simulink model "Autopilot_q_full_5may_new1"  (R2020a)
settings: Solver=ode4  StartTime=0.0  StopTime=300  FixedStep=0.01  RelTol=1e-3
undefined symbols (not defined in the file or in its folder): Aero_cofficients, Atmosphere_pert, Atmospheric_model, Counter_sensor_model, Earth, error_global, flags_global, Guidance_Flags_global, INT_global, param_guidance, Payload_data, Plane_state_mode_finish_catcher_ftr_mode, Plane_state_mode_finish_catcher_fw_mode, Plane_state_mode_finish_catcher_q_mode, Plane_state_mode_finish_catcher_rtr_mode, Plane_state_store, propulsion_model, propulsion_model_int, Structural_data, Thrust_data_store, time_global, WGS84, Wind_data, Wind_model_int, Wind_pert_factor
libraries: simulink x33, aerolibactuator x15, cstblocks x3, aerolibatmos2 x2, aerolibfltsims x1, aerolibtransform2 x1, shared6dof x1
(part 4 of 10)

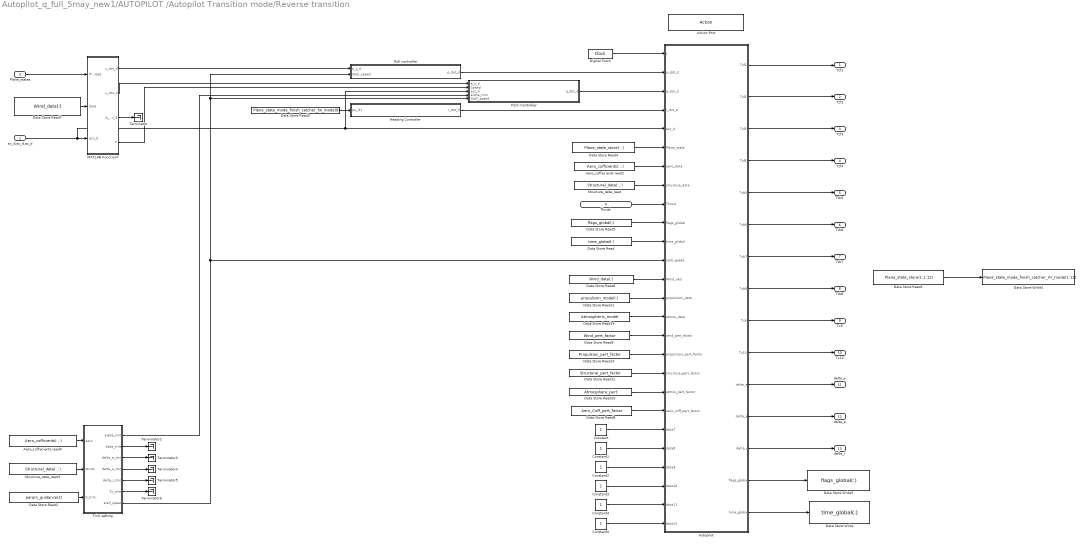
== system Autopilot_q_full_5may_new1/AUTOPILOT /Autopilot Transition mode/Reverse transition ==
  ax_d,ay_d,az_d : Inport
  Plane_states : Inport  Port=2
  Thrust : Inport  Port=3
  Action Port : ActionPort  ActionPortLabel=if { }
  Aero_coffecients read2 : DataStoreRead  Priority=1  DataStoreName=Aero_cofficients  DataStoreElements=Aero_cofficients(:,:)
  Aero_coffecients read4 : DataStoreRead  DataStoreName=Aero_cofficients  DataStoreElements=Aero_cofficients(:,:)
  Autopilot : MATLAB Function  TreatAsAtomicUnit=on
  Constant{,1..5} (6 alike) : Constant
  Data Store Read : DataStoreRead  DataStoreName=time_global  DataStoreElements=time_global(:)
  Data Store Read1 : DataStoreRead  DataStoreName=Plane_state_store  DataStoreElements=Plane_state_store(1,1:12)
  Data Store Read10 : DataStoreRead  DataStoreName=Atmosphere_pert
  Data Store Read11 : DataStoreRead  DataStoreName=propulsion_model  DataStoreElements=propulsion_model(:)
  Data Store Read12 : DataStoreRead  DataStoreName=Structural_pert_factor
  Data Store Read13 : DataStoreRead  DataStoreName=Propulsion_pert_factor
  Data Store Read14 : DataStoreRead  DataStoreName=Atmospheric_model
  Data Store Read2 : DataStoreRead  DataStoreName=param_guidance  DataStoreElements=param_guidance(2)
  Data Store Read3 : DataStoreRead  DataStoreName=Plane_state_mode_finish_catcher_fw_mode  DataStoreElements=Plane_state_mode_finish_catcher_fw_mode(9)
  Data Store Read4 : DataStoreRead  DataStoreName=Plane_state_store  DataStoreElements=Plane_state_store(:,:)
  Data Store Read5 : DataStoreRead  DataStoreName=flags_global  DataStoreElements=flags_global(:)
  Data Store Read6 : DataStoreRead  DataStoreName=Wind_data  DataStoreElements=Wind_data(:)
  Data Store Read7 : DataStoreRead  DataStoreName=Wind_data  DataStoreElements=Wind_data(:)
  Data Store Read8 : DataStoreRead  DataStoreName=Aero_Coff_pert_factor
  Data Store Read9 : DataStoreRead  DataStoreName=Wind_pert_factor
  Data Store Write : DataStoreWrite  DataStoreName=time_global  DataStoreElements=time_global(:)
  Data Store Write1 : DataStoreWrite  DataStoreName=Plane_state_mode_finish_catcher_rtr_mode  DataStoreElements=Plane_state_mode_finish_catcher_rtr_mode(1:12)
  Data Store Write5 : DataStoreWrite  DataStoreName=flags_global  DataStoreElements=flags_global(:)
  Digital Clock : DigitalClock  SampleTime=0.01
  Heading Controller : Subsystem
  MATLAB Function7 : MATLAB Function  TreatAsAtomicUnit=on
  Pitch Controller : Subsystem
  Roll controller : Subsystem
  Structure_data_read : DataStoreRead  Priority=2  DataStoreName=Structural_data  DataStoreElements=Structural_data(:,:)
  Structure_data_read3 : DataStoreRead  DataStoreName=Structural_data  DataStoreElements=Structural_data(:,:)
  Terminator{,2..6} (6 alike) : Terminator
  Trim setting : Subsystem
  Tzf1 : Outport  VectorParamsAs1DForOutWhenUnconnected=off
  Tzf2 : Outport  Port=2  VectorParamsAs1DForOutWhenUnconnected=off
  Tzf3 : Outport  Port=3  VectorParamsAs1DForOutWhenUnconnected=off
  Tzf4 : Outport  Port=4  VectorParamsAs1DForOutWhenUnconnected=off
  Tzb5 : Outport  Port=5  VectorParamsAs1DForOutWhenUnconnected=off
  Tzb6 : Outport  Port=6  VectorParamsAs1DForOutWhenUnconnected=off
  Tzb7 : Outport  Port=7  VectorParamsAs1DForOutWhenUnconnected=off
  Tzb8 : Outport  Port=8  VectorParamsAs1DForOutWhenUnconnected=off
  Tx9 : Outport  Port=9  VectorParamsAs1DForOutWhenUnconnected=off
  Tx10 : Outport  Port=10  VectorParamsAs1DForOutWhenUnconnected=off
  delta_e : Outport  Port=11  VectorParamsAs1DForOutWhenUnconnected=off
  delta_a : Outport  Port=12  VectorParamsAs1DForOutWhenUnconnected=off
  delta_r : Outport  Port=13  VectorParamsAs1DForOutWhenUnconnected=off
  wires:
  Autopilot/12(delta_a) -> delta_a/1
  MATLAB Function7/3(w_dot_d) -> Terminator/1
  Autopilot/10(Tx10) -> Tx10/1
  Roll controller/1(p_dot_d) -> Autopilot/2(p_dot_d)
  Autopilot/4(Tzf4) -> Tzf4/1
  Autopilot/1(Tzf1) -> Tzf1/1
  Autopilot/8(Tzb8) -> Tzb8/1
  Trim setting/6(Tx_trim) -> Terminator6/1
  Trim setting/2(beta_trim) -> Terminator2/1
  Heading Controller/1(r_dot_d) -> Autopilot/4(r_dot_d)
  Trim setting/3(delta_e_trim) -> Terminator3/1
  Structure_data_read3/1 -> Trim setting/2("struct ")
  Trim setting/5(delta_r_trim) -> Terminator5/1
  Autopilot/2(Tzf2) -> Tzf2/1
  Autopilot/5(Tzb5) -> Tzb5/1
  ax_d,ay_d,az_d/1 -> Pitch Controller/3(acc_d), Autopilot/5(acc_d), MATLAB Function7/3(acc_d)
  Autopilot/9(Tx9) -> Tx9/1
  Data Store Read2/1 -> Trim setting/3(V_trim)
  Autopilot/11(delta_e) -> delta_e/1
  Autopilot/6(Tzb6) -> Tzb6/1
  Autopilot/3(Tzf3) -> Tzf3/1
  Autopilot/13(delta_r) -> delta_r/1
  Aero_coffecients read4/1 -> Trim setting/1("aero ")
  Autopilot/7(Tzb7) -> Tzb7/1
  Trim setting/4(delta_a_trim) -> Terminator4/1
  Trim setting/7(stall_speed) -> Roll controller/2(Stall_speed), Pitch Controller/5(Stall_speed), Autopilot/12(stall_speed)
  Autopilot/14(flags_global) -> Data Store Write5/1
  Data Store Read5/1 -> Autopilot/10("flags_global ")
  Autopilot/15(time_global) -> Data Store Write/1
  Data Store Read/1 -> Autopilot/11("time_global ")
  Digital Clock/1 -> Autopilot/1(t)
  Data Store Read1/1 -> Data Store Write1/1
  Pitch Controller/1(q_dot_d) -> Autopilot/3(q_dot_d)
  Aero_coffecients read2/1 -> Autopilot/7(aero_data)
  Structure_data_read/1 -> Autopilot/8(structure_data)
  Thrust/1 -> Autopilot/9(Thrust)
  MATLAB Function7/1(v_dot_d) -> Roll controller/1(a_y_d)
  MATLAB Function7/2(u_dot_d) -> Pitch Controller/1(a_x_d)
  Trim setting/1(alpha_trim) -> Pitch Controller/4(alpha_trim)
  Data Store Read3/1 -> Heading Controller/1(psi_d1)
  MATLAB Function7/4(V) -> Pitch Controller/2(Speed)
  Data Store Read4/1 -> Autopilot/6(Plane_state)
  Data Store Read6/1 -> Autopilot/13(Wind_ned)
  Data Store Read7/1 -> MATLAB Function7/2(data)
  Plane_states/1 -> MATLAB Function7/1(Plane_state)
  Data Store Read11/1 -> Autopilot/14(propulsion_data)
  Data Store Read14/1 -> Autopilot/15(atmos_data)
  Data Store Read9/1 -> Autopilot/16(wind_pert_factor)
  Data Store Read13/1 -> Autopilot/17(propulsion_pert_factor)
  Data Store Read12/1 -> Autopilot/18(structure_pert_factor)
  Data Store Read10/1 -> Autopilot/19(atmos_pert_factor)
  Data Store Read8/1 -> Autopilot/20(aero_coff_pert_factor)
  Constant/1 -> Autopilot/21(data7)
  Constant1/1 -> Autopilot/22(data8)
  Constant2/1 -> Autopilot/23(data9)
  Constant3/1 -> Autopilot/24(data10)
  Constant4/1 -> Autopilot/25(data11)
  Constant5/1 -> Autopilot/26(data12)

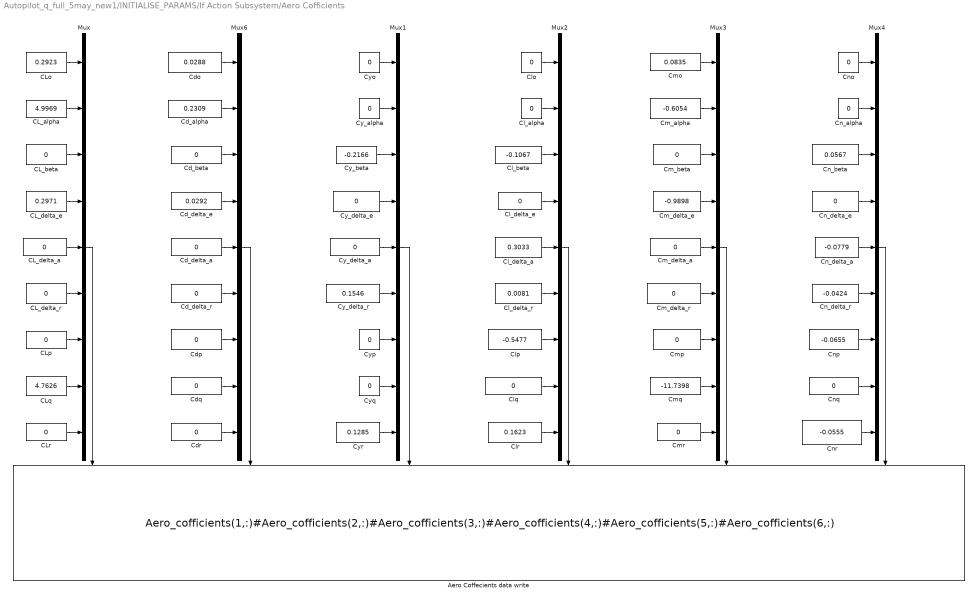
== system Autopilot_q_full_5may_new1/INITIALISE_PARAMS/If Action Subsystem/Aero Cofficients ==
  Aero Coffecients data write : DataStoreWrite  DataStoreName=Aero_cofficients  DataStoreElements=Aero_cofficients(1,:)#Aero_cofficients(2,:)#Aero_cofficients(3,:)#Aero_cofficients(4,:)#Aero_cofficients(5,:)#Aero_cofficients(6,:)
  CL_alpha : Constant  Value=4.9969
  CL_beta : Constant  Value=0
  CL_delta_a : Constant  Value=0
  CL_delta_e : Constant  Value=0.2971
  CL_delta_r : Constant  Value=0
  CLo : Constant  Value=0.2923
  CLp : Constant  Value=0
  CLq : Constant  Value=4.7626
  CLr : Constant  Value=0
  Cd_alpha : Constant  Value=0.2309
  Cd_beta : Constant  Value=0
  Cd_delta_a : Constant  Value=0
  Cd_delta_e : Constant  Value=0.0292
  Cd_delta_r : Constant  Value=0
  Cdo : Constant  Value=0.0288
  Cdp : Constant  Value=0
  Cdq : Constant  Value=0
  Cdr : Constant  Value=0
  Cl_alpha : Constant  Value=0
  Cl_beta : Constant  Value=-0.1067
  Cl_delta_a : Constant  Value=0.3033
  Cl_delta_e : Constant  Value=0
  Cl_delta_r : Constant  Value=0.0081
  Clo : Constant  Value=0
  Clp : Constant  Value=-0.5477
  Clq : Constant  Value=0
  Clr : Constant  Value=0.1623
  Cm_alpha : Constant  Value=-0.6054
  Cm_beta : Constant  Value=0
  Cm_delta_a : Constant  Value=0
  Cm_delta_e : Constant  Value=-0.9898
  Cm_delta_r : Constant  Value=0
  Cmo : Constant  Value=0.0835
  Cmp : Constant  Value=0
  Cmq : Constant  Value=-11.7398
  Cmr : Constant  Value=0
  Cn_alpha : Constant  Value=0
  Cn_beta : Constant  Value=0.0567
  Cn_delta_a : Constant  Value=-0.0779
  Cn_delta_e : Constant  Value=0
  Cn_delta_r : Constant  Value=-0.0424
  Cno : Constant  Value=0
  Cnp : Constant  Value=-0.0655
  Cnq : Constant  Value=0
  Cnr : Constant  Value=-0.0555
  Cy_alpha : Constant  Value=0
  Cy_beta : Constant  Value=-0.2166
  Cy_delta_a : Constant  Value=0
  Cy_delta_e : Constant  Value=0
  Cy_delta_r : Constant  Value=0.1546
  Cyo : Constant  Value=0
  Cyp : Constant  Value=0
  Cyq : Constant  Value=0
  Cyr : Constant  Value=0.1285
  Mux{,1..4,6} (6 alike) : Mux  Inputs=9
  wires:
  Mux/1 -> Aero Coffecients data write/1
  Cl_delta_a/1 -> Mux2/5
  Cyq/1 -> Mux1/8
  CL_beta/1 -> Mux/3
  Cdo/1 -> Mux6/1
  Cm_beta/1 -> Mux3/3
  Cy_beta/1 -> Mux1/3
  Cy_delta_e/1 -> Mux1/4
  Cm_delta_e/1 -> Mux3/4
  CLr/1 -> Mux/9
  Cnp/1 -> Mux4/7
  Cyp/1 -> Mux1/7
  CLo/1 -> Mux/1
  Cy_alpha/1 -> Mux1/2
  Cdp/1 -> Mux6/7
  CLq/1 -> Mux/8
  Cl_alpha/1 -> Mux2/2
  Cmq/1 -> Mux3/8
  Mux3/1 -> Aero Coffecients data write/5
  Cnq/1 -> Mux4/8
  Cn_delta_r/1 -> Mux4/6
  Cn_beta/1 -> Mux4/3
  Cdr/1 -> Mux6/9
  Clr/1 -> Mux2/9
  Cd_delta_a/1 -> Mux6/5
  Clq/1 -> Mux2/8
  Cn_delta_e/1 -> Mux4/4
  Clo/1 -> Mux2/1
  Cy_delta_r/1 -> Mux1/6
  Cnr/1 -> Mux4/9
  Cm_delta_r/1 -> Mux3/6
  Cyo/1 -> Mux1/1
  CL_delta_a/1 -> Mux/5
  Clp/1 -> Mux2/7
  Mux2/1 -> Aero Coffecients data write/4
  Cmp/1 -> Mux3/7
  Mux1/1 -> Aero Coffecients data write/3
  CL_delta_r/1 -> Mux/6
  Mux6/1 -> Aero Coffecients data write/2
  Cl_delta_r/1 -> Mux2/6
  Cdq/1 -> Mux6/8
  CL_delta_e/1 -> Mux/4
  Cl_beta/1 -> Mux2/3
  Cd_delta_r/1 -> Mux6/6
  Cmo/1 -> Mux3/1
  Cno/1 -> Mux4/1
  Cmr/1 -> Mux3/9
  Cyr/1 -> Mux1/9
  Cn_delta_a/1 -> Mux4/5
  Cl_delta_e/1 -> Mux2/4
  Cd_delta_e/1 -> Mux6/4
  Cd_alpha/1 -> Mux6/2
  Cm_delta_a/1 -> Mux3/5
  Cn_alpha/1 -> Mux4/2
  Cm_alpha/1 -> Mux3/2
  Cd_beta/1 -> Mux6/3
  Mux4/1 -> Aero Coffecients data write/6
  CLp/1 -> Mux/7
  CL_alpha/1 -> Mux/2
  Cy_delta_a/1 -> Mux1/5

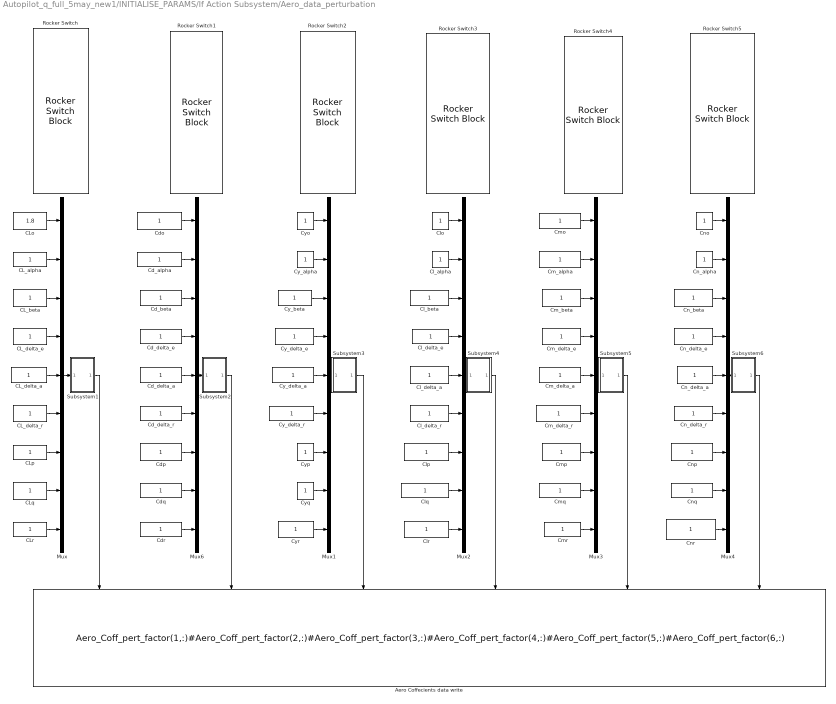
== system Autopilot_q_full_5may_new1/INITIALISE_PARAMS/If Action Subsystem/Aero_data_perturbation ==
  Aero Coffecients data write : DataStoreWrite  DataStoreName=Aero_Coff_pert_factor  DataStoreElements=Aero_Coff_pert_factor(1,:)#Aero_Coff_pert_factor(2,:)#Aero_Coff_pert_factor(3,:)#Aero_Coff_pert_factor(4,:)#Aero_Coff_pert_factor(5,:)#Aero_Coff_pert_factor(6,:)
  CL_alpha : Constant
  CL_beta : Constant
  CL_delta_a : Constant
  CL_delta_e : Constant
  CL_delta_r : Constant
  CLo : Constant  Value=1.8
  CLp : Constant
  CLq : Constant
  CLr : Constant
  Cd_alpha : Constant
  Cd_beta : Constant
  Cd_delta_a : Constant
  Cd_delta_e : Constant
  Cd_delta_r : Constant
  Cdo : Constant
  Cdp : Constant
  Cdq : Constant
  Cdr : Constant
  Cl_alpha : Constant
  Cl_beta : Constant
  Cl_delta_a : Constant
  Cl_delta_e : Constant
  Cl_delta_r : Constant
  Clo : Constant
  Clp : Constant
  Clq : Constant
  Clr : Constant
  Cm_alpha : Constant
  Cm_beta : Constant
  Cm_delta_a : Constant
  Cm_delta_e : Constant
  Cm_delta_r : Constant
  Cmo : Constant
  Cmp : Constant
  Cmq : Constant
  Cmr : Constant
  Cn_alpha : Constant
  Cn_beta : Constant
  Cn_delta_a : Constant
  Cn_delta_e : Constant
  Cn_delta_r : Constant
  Cno : Constant
  Cnp : Constant
  Cnq : Constant
  Cnr : Constant
  Cy_alpha : Constant
  Cy_beta : Constant
  Cy_delta_a : Constant
  Cy_delta_e : Constant
  Cy_delta_r : Constant
  Cyo : Constant
  Cyp : Constant
  Cyq : Constant
  Cyr : Constant
  Mux{,1..4,6} (6 alike) : Mux  Inputs=9
  Rocker Switch{,1..5} (6 alike) : RockerSwitchBlock
      settings: Values={{'Off', 'On'}, [0 1]}
  Subsystem1 : Subsystem
  Subsystem2 : Subsystem
  Subsystem3 : Subsystem
  Subsystem4 : Subsystem
  Subsystem5 : Subsystem
  Subsystem6 : Subsystem
  wires:
  CL_delta_e/1 -> Mux/4
  Cdp/1 -> Mux6/7
  Cd_alpha/1 -> Mux6/2
  Cn_delta_a/1 -> Mux4/5
  Cn_delta_e/1 -> Mux4/4
  Cmr/1 -> Mux3/9
  Cn_delta_r/1 -> Mux4/6
  Cd_delta_a/1 -> Mux6/5
  Cl_delta_e/1 -> Mux2/4
  Cd_beta/1 -> Mux6/3
  Cm_delta_a/1 -> Mux3/5
  Cd_delta_r/1 -> Mux6/6
  Cyr/1 -> Mux1/9
  Cdo/1 -> Mux6/1
  Cm_delta_e/1 -> Mux3/4
  Cyo/1 -> Mux1/1
  Cmp/1 -> Mux3/7
  Cdq/1 -> Mux6/8
  CL_delta_r/1 -> Mux/6
  Cmq/1 -> Mux3/8
  Cy_beta/1 -> Mux1/3
  Clp/1 -> Mux2/7
  CLo/1 -> Mux/1
  Cy_delta_a/1 -> Mux1/5
  CLq/1 -> Mux/8
  Cl_delta_r/1 -> Mux2/6
  CL_alpha/1 -> Mux/2
  Cnp/1 -> Mux4/7
  Cm_alpha/1 -> Mux3/2
  Cy_delta_e/1 -> Mux1/4
  Clr/1 -> Mux2/9
  Cy_alpha/1 -> Mux1/2
  Cnq/1 -> Mux4/8
  Cyp/1 -> Mux1/7
  Cnr/1 -> Mux4/9
  CLp/1 -> Mux/7
  Clq/1 -> Mux2/8
  CL_delta_a/1 -> Mux/5
  Cno/1 -> Mux4/1
  Cl_alpha/1 -> Mux2/2
  Cm_delta_r/1 -> Mux3/6
  Clo/1 -> Mux2/1
  Cdr/1 -> Mux6/9
  Cd_delta_e/1 -> Mux6/4
  Cl_delta_a/1 -> Mux2/5
  CL_beta/1 -> Mux/3
  Cmo/1 -> Mux3/1
  CLr/1 -> Mux/9
  Cyq/1 -> Mux1/8
  Cl_beta/1 -> Mux2/3
  Cy_delta_r/1 -> Mux1/6
  Cm_beta/1 -> Mux3/3
  Cn_beta/1 -> Mux4/3
  Cn_alpha/1 -> Mux4/2
  Mux/1 -> Subsystem1/1(In1)
  Subsystem1/1(Out1) -> Aero Coffecients data write/1
  Mux6/1 -> Subsystem2/1(In1)
  Subsystem2/1(Out1) -> Aero Coffecients data write/2
  Mux1/1 -> Subsystem3/1(In1)
  Mux2/1 -> Subsystem4/1(In1)
  Mux3/1 -> Subsystem5/1(In1)
  Mux4/1 -> Subsystem6/1(In1)
  Subsystem3/1(Out1) -> Aero Coffecients data write/3
  Subsystem4/1(Out1) -> Aero Coffecients data write/4
  Subsystem5/1(Out1) -> Aero Coffecients data write/5
  Subsystem6/1(Out1) -> Aero Coffecients data write/6

== system Autopilot_q_full_5may_new1/INITIALISE_PARAMS/If Action Subsystem/Atmosphere_pert ==
  note: Temp
  note: density
  note: a
  note: p
  Constant{,1..3} (4 alike) : Constant
  Data Store Write : DataStoreWrite  DataStoreName=Atmosphere_pert  DataStoreElements=Atmosphere_pert(:)
  Mux : Mux
  Rocker Switch : RockerSwitchBlock
      settings: Values={{'Off', 'On'}, [0 1]}
  Subsystem1 : Subsystem
  wires:
  Subsystem1/1(Out1) -> Data Store Write/1
  Constant/1 -> Mux/1
  Mux/1 -> Subsystem1/1(In1)
  Constant1/1 -> Mux/2
  Constant2/1 -> Mux/3
  Constant3/1 -> Mux/4

== system Autopilot_q_full_5may_new1/INITIALISE_PARAMS/If Action Subsystem/Atmospheric model ==
  Abs : Abs
  Constant : Constant  Value=0.1
  Data Store Write : DataStoreWrite  DataStoreName=Atmospheric_model  DataStoreElements=Atmospheric_model(:)
  ISA Atmosphere Model : aerolibatmos2/ISA Atmosphere Model  custom=off  g=9.80665  gamma=1.4  R=287.0531  L=0.0065  h_trop=11000  h_strat=20000  rho0=1.225  P0=101325  T0=288.15  h0=0
  Mux : Mux
  Scope{1..2,4..5} (4 alike) : Scope
  wires:
  ISA Atmosphere Model/4 -> Scope2/1, Mux/4
  ISA Atmosphere Model/1 -> Scope1/1, Mux/1
  ISA Atmosphere Model/2 -> Mux/2, Scope4/1
  ISA Atmosphere Model/3 -> Mux/3, Scope5/1
  Abs/1 -> ISA Atmosphere Model/1
  Mux/1 -> Data Store Write/1
  Constant/1 -> Abs/1

== system Autopilot_q_full_5may_new1/INITIALISE_PARAMS/If Action Subsystem/INT_global ==
  INT_GLOBAL : DataStoreWrite  DataStoreName=INT_global  DataStoreElements=INT_global(1)#INT_global(2)#INT_global(3)#INT_global(4)#INT_global(5)#INT_global(6)#INT_global(7)#INT_global(8)#INT_global(9)#INT_global(10)#INT_global(11)#INT_global(12)#INT_global(13)#INT_global(14)
  INT_VX : Constant  Value=0
  INT_VY : Constant  Value=0
  INT_VZ : Constant  Value=0
  INT_X : Constant  Value=0
  INT_Y : Constant  Value=0
  INT_Z : Constant  Value=0
  INT_alpha : Constant  Value=0
  INT_beta : Constant  Value=0
  INT_p : Constant  Value=0
  INT_phi : Constant  Value=0
  INT_psi : Constant  Value=0
  INT_q : Constant  Value=0
  INT_r : Constant  Value=0
  INT_theta : Constant  Value=0
  wires:
  INT_VX/1 -> INT_GLOBAL/4
  INT_r/1 -> INT_GLOBAL/12
  INT_Y/1 -> INT_GLOBAL/2
  INT_q/1 -> INT_GLOBAL/11
  INT_beta/1 -> INT_GLOBAL/14
  INT_Z/1 -> INT_GLOBAL/3
  INT_VZ/1 -> INT_GLOBAL/6
  INT_phi/1 -> INT_GLOBAL/7
  INT_X/1 -> INT_GLOBAL/1
  INT_p/1 -> INT_GLOBAL/10
  INT_VY/1 -> INT_GLOBAL/5
  INT_theta/1 -> INT_GLOBAL/8
  INT_alpha/1 -> INT_GLOBAL/13
  INT_psi/1 -> INT_GLOBAL/9

== system Autopilot_q_full_5may_new1/INITIALISE_PARAMS/If Action Subsystem/Params ==
  Cruise_speed : Constant  Value=25
  lim_pos : Constant  Value=0.001
  lim_vel : Constant  Value=0.001
  loiter radius : Constant  Value=60
  time store write 1 : DataStoreWrite  DataStoreName=param_guidance  DataStoreElements=param_guidance(1)#param_guidance(2)#param_guidance(3)#param_guidance(4)
  wires:
  Cruise_speed/1 -> time store write 1/2
  loiter radius/1 -> time store write 1/1
  lim_vel/1 -> time store write 1/4
  lim_pos/1 -> time store write 1/3

== system Autopilot_q_full_5may_new1/INITIALISE_PARAMS/If Action Subsystem/Payload_data ==
  note: Payload Model on off
  Constant : Constant  Value=0
  Data Store Write : DataStoreWrite  DataStoreName=Payload_data  DataStoreElements=Payload_data(1)
  Rocker Switch : RockerSwitchBlock
      settings: Values={{'Off', 'On'}, [0 1]}
  wires:
  Constant/1 -> Data Store Write/1

== system Autopilot_q_full_5may_new1/INITIALISE_PARAMS/If Action Subsystem/Propulsion_Model ==
  Data Store Write : DataStoreWrite  DataStoreName=propulsion_model_int  DataStoreElements=propulsion_model_int(:)
  Data Store Write1 : DataStoreWrite  DataStoreName=propulsion_model  DataStoreElements=propulsion_model(:)
  Mux : Mux
  PUSHER Propeller drag factor : Constant  Value=1.9899*10^-8
  PUSHER Propeller thrust factor : Constant  Value=6.679*10^-7
  VTOL Propeller drag factor : Constant  Value=1.8928*10^-8
  VTOL Propeller thrust factor : Constant  Value=5.6143*10^-7
  wires:
  VTOL Propeller thrust factor/1 -> Mux/1
  VTOL Propeller drag factor/1 -> Mux/2
  Mux/1 -> Data Store Write1/1, Data Store Write/1
  PUSHER Propeller thrust factor/1 -> Mux/3
  PUSHER Propeller drag factor/1 -> Mux/4

== system Autopilot_q_full_5may_new1/INITIALISE_PARAMS/If Action Subsystem/Propulsion_data_pert ==
  note: b_vtol
  note: d_vtol
  note: d_pusher
  note: b_pusher
  Constant{,1..3} (4 alike) : Constant
  Data Store Write : DataStoreWrite  DataStoreName=Propulsion_pert_factor  DataStoreElements=Propulsion_pert_factor(1:2)#Propulsion_pert_factor(3:4)
  Mux : Mux  Inputs=2
  Mux1 : Mux  Inputs=2
  Rocker Switch : RockerSwitchBlock
      settings: Values={{'Off', 'On'}, [0 1]}
  Rocker Switch1 : RockerSwitchBlock
      settings: Values={{'Off', 'On'}, [0 1]}
  Subsystem1 : Subsystem
  Subsystem2 : Subsystem
  wires:
  Constant/1 -> Mux/1
  Mux/1 -> Subsystem1/1(In1)
  Constant1/1 -> Mux/2
  Subsystem1/1(Out1) -> Data Store Write/1
  Constant3/1 -> Mux1/2
  Mux1/1 -> Subsystem2/1(In1)
  Constant2/1 -> Mux1/1
  Subsystem2/1(Out1) -> Data Store Write/2

== system Autopilot_q_full_5may_new1/INITIALISE_PARAMS/If Action Subsystem/Structure_data ==
  Ixx : Constant  Value=0.6275
  Ixy : Constant  Value=0
  Ixz : Constant  Value=0
  Iyy : Constant  Value=0.564
  Iyz : Constant  Value=0
  Izz : Constant  Value=1.176
  Mass : Constant  Value=5
  Structure data write1 : DataStoreWrite  DataStoreName=Structural_data  DataStoreElements=Structural_data(1,1)#Structural_data(1,2)#Structural_data(1,3)#Structural_data(1,4)#Structural_data(1,5)#Structural_data(1,6)#Structural_data(1,7)#Structural_data(1,8)#Structural_data(1,9)#Structural_data(1,10)#Structural_data(1,11)#Structural_data(1,12)#Structural_data(1,13)#Structural_data(1,14)#Structural_data(1,15)#Structural_data(1,16)#Structural_data(1,17)#Structural_data(1,18)#Structural_data(1,19)#Structural_data(1,20)#Structural_data(1,21)#Structural_data(1,22)#Structural_data(1,23)#Structural_data(1,24)
  b : Constant  Value=2.2
  c : Constant  Value=0.2104
  mb : Constant  Value=0
  s : Constant  Value=0.4626
  x1 : Constant  Value=743/2000
  x2 : Constant  Value=-743/2000
  y1 : Constant  Value=-838/1000
  y10 : Constant  Value=0
  y2 : Constant  Value=-838/2000
  y3 : Constant  Value=838/2000
  y4 : Constant  Value=838/1000
  y5 : Constant  Value=-838/1000
  y6 : Constant  Value=-838/2000
  y7 : Constant  Value=838/2000
  y8 : Constant  Value=838/1000
  y9 : Constant  Value=0.0
  z1 : Constant  Value=0
  wires:
  y5/1 -> Structure data write1/17
  Ixz/1 -> Structure data write1/9
  y6/1 -> Structure data write1/18
  y3/1 -> Structure data write1/15
  s/1 -> Structure data write1/4
  b/1 -> Structure data write1/3
  z1/1 -> Structure data write1/23
  y8/1 -> Structure data write1/20
  Mass/1 -> Structure data write1/1
  x2/1 -> Structure data write1/12
  y2/1 -> Structure data write1/14
  y10/1 -> Structure data write1/22
  y9/1 -> Structure data write1/21
  Iyy/1 -> Structure data write1/6
  c/1 -> Structure data write1/2
  mb/1 -> Structure data write1/24
  Ixx/1 -> Structure data write1/5
  x1/1 -> Structure data write1/11
  y4/1 -> Structure data write1/16
  Iyz/1 -> Structure data write1/10
  Izz/1 -> Structure data write1/7
  y7/1 -> Structure data write1/19
  Ixy/1 -> Structure data write1/8
  y1/1 -> Structure data write1/13

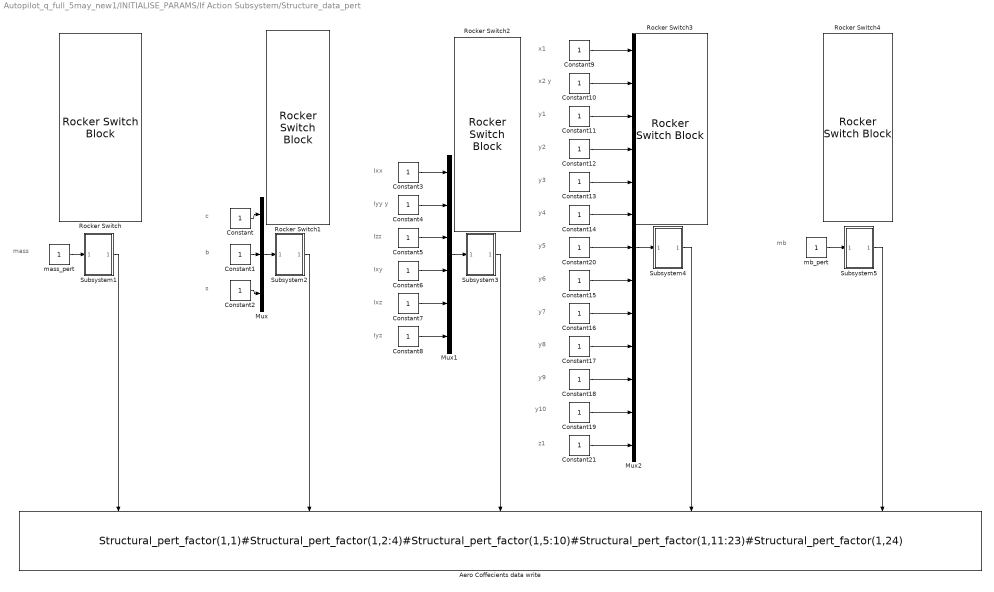
== system Autopilot_q_full_5may_new1/INITIALISE_PARAMS/If Action Subsystem/Structure_data_pert ==
  note: c
  note: b
  note: s
  note: Ixx
  note: Iyy y
  note: Izz
  note: Ixy
  note: Ixz
  note: Iyz
  note: mass
  note: y4
  note: y2
  note: y3
  note: x2 y
  note: x1
  note: y1
  note: y6
  note: y7
  note: y8
  note: y5
  note: z1
  note: y10
  note: y9
  note: mb
  Aero Coffecients data write : DataStoreWrite  DataStoreName=Structural_pert_factor  DataStoreElements=Structural_pert_factor(1,1)#Structural_pert_factor(1,2:4)#Structural_pert_factor(1,5:10)#Structural_pert_factor(1,11:23)#Structural_pert_factor(1,24)
  Constant{,1..21} (22 alike) : Constant
  Mux : Mux  Inputs=3
  Mux1 : Mux  Inputs=6
  Mux2 : Mux  Inputs=13
  Rocker Switch{,1..4} (5 alike) : RockerSwitchBlock
      settings: Values={{'Off', 'On'}, [0 1]}
  Subsystem1 : Subsystem
  Subsystem2 : Subsystem
  Subsystem3 : Subsystem
  Subsystem4 : Subsystem
  Subsystem5 : Subsystem
  mass_pert : Constant
  mb_pert : Constant
  wires:
  Mux1/1 -> Subsystem3/1(In1)
  Subsystem1/1(Out1) -> Aero Coffecients data write/1
  Subsystem5/1(Out1) -> Aero Coffecients data write/5
  Subsystem4/1(Out1) -> Aero Coffecients data write/4
  Subsystem3/1(Out1) -> Aero Coffecients data write/3
  Subsystem2/1(Out1) -> Aero Coffecients data write/2
  mass_pert/1 -> Subsystem1/1(In1)
  Mux/1 -> Subsystem2/1(In1)
  Constant/1 -> Mux/1
  Constant1/1 -> Mux/2
  Constant2/1 -> Mux/3
  Constant3/1 -> Mux1/1
  Constant4/1 -> Mux1/2
  Constant5/1 -> Mux1/3
  Constant6/1 -> Mux1/4
  Constant7/1 -> Mux1/5
  Constant8/1 -> Mux1/6
  Constant14/1 -> Mux2/6
  Constant9/1 -> Mux2/1
  Constant13/1 -> Mux2/5
  Constant11/1 -> Mux2/3
  Constant10/1 -> Mux2/2
  Constant12/1 -> Mux2/4
  Mux2/1 -> Subsystem4/1(In1)
  Constant20/1 -> Mux2/7
  Constant17/1 -> Mux2/10
  Constant15/1 -> Mux2/8
  Constant16/1 -> Mux2/9
  Constant19/1 -> Mux2/12
  Constant18/1 -> Mux2/11
  mb_pert/1 -> Subsystem5/1(In1)
  Constant21/1 -> Mux2/13

== system Autopilot_q_full_5may_new1/INITIALISE_PARAMS/If Action Subsystem/Time_global ==
  note: Initial lift off hover
  note: Vertical lift off
  note: Hover
  note: Cruise/Loiter , All fixed wing here
  note: Reverse Transition
  note: Hover
  note: Vertical Landing
  note: Forward Transition
  tf0 : Constant  Value=0
  tf1 : Constant  Value=0
  tf2 : Constant  Value=20
  tf3 : Constant  Value=22
  tf4 : Constant  Value=30
  tf5 : Constant  Value=50
  tf6 : Constant  Value=70
  tf7 : Constant  Value=72
  tf8 : Constant  Value=92
  "time store write " : DataStoreWrite  DataStoreName=time_global  DataStoreElements=time_global(1)#time_global(2)#time_global(3)#time_global(4)#time_global(5)#time_global(6)#time_global(7)#time_global(8)#time_global(9)
  wires:
  tf4/1 -> "time store write "/5
  tf8/1 -> "time store write "/9
  tf1/1 -> "time store write "/2
  tf6/1 -> "time store write "/7
  tf2/1 -> "time store write "/3
  tf5/1 -> "time store write "/6
  tf0/1 -> "time store write "/1
  tf7/1 -> "time store write "/8
  tf3/1 -> "time store write "/4

== system Autopilot_q_full_5may_new1/INITIALISE_PARAMS/If Action Subsystem/Wind_Model ==
  note: turb_on_off<50 m
  note: VN
  note: VE
  note: VD
  note: turb_on_off- 50-600 m
  note: turb_on_off>600 m
  note: turb_on_off<50 m
  note: turb_on_off- 50-600 m
  note: turb_on_off>600 m
  Constant4 : Constant  Value=0
  Constant5 : Constant  Value=0
  Constant6 : Constant  Value=0
  Data Store Write : DataStoreWrite  DataStoreName=Wind_model_int  DataStoreElements=Wind_model_int(1:3)
  Data Store Write1 : DataStoreWrite  DataStoreName=Wind_model_int  DataStoreElements=Wind_model_int(4:10)
  Moderate_turbulence_50 : RockerSwitchBlock
      settings: Values={{'Off', 'On'}, [0 1]}
  Mux : Mux  Inputs=3
  Mux1 : Mux  Inputs=7
  Rocker Switch : RockerSwitchBlock
      settings: Values={{'Off', 'On'}, [0 1]}
  Rocker Switch1 : RockerSwitchBlock
      settings: Values={{'Off', 'On'}, [0 1]}
  Rocker Switch2 : RockerSwitchBlock
      settings: Values={{'Off', 'On'}, [0 1]}
  light_turb_2 : Constant  Value=0
  light_turb_50 : Constant
  light_turb_600 : Constant
  light_turbulence_50 : RockerSwitchBlock
      settings: Values={{'Off', 'On'}, [0 1]}
  light_turbulence_600 : RockerSwitchBlock
      settings: Values={{'Off', 'On'}, [0 1]}
  mod_turb_50 : Constant  Value=0
  mod_turb_600 : Constant  Value=0
  moderate_turbulence_600 : RockerSwitchBlock
      settings: Values={{'Off', 'On'}, [0 1]}
  turb_50 : Constant  Value=0
  turb_50_600 : Constant  Value=0
  wires:
  Constant4/1 -> Mux/1
  Constant5/1 -> Mux/2
  Constant6/1 -> Mux/3
  Mux/1 -> Data Store Write/1
  light_turb_600/1 -> Mux1/3
  light_turb_50/1 -> Mux1/1
  mod_turb_50/1 -> Mux1/2
  mod_turb_600/1 -> Mux1/4
  Mux1/1 -> Data Store Write1/1
  turb_50_600/1 -> Mux1/6
  light_turb_2/1 -> Mux1/7
  turb_50/1 -> Mux1/5

== system Autopilot_q_full_5may_new1/INITIALISE_PARAMS/If Action Subsystem/Wind_data_pert ==
  note: V_N
  note: V_E
  note: V_D
  Constant : Constant
  Constant1 : Constant
  Constant2 : Constant
  Data Store Write : DataStoreWrite  DataStoreName=Wind_pert_factor  DataStoreElements=Wind_pert_factor(:)
  Mux : Mux  Inputs=3
  Rocker Switch : RockerSwitchBlock
      settings: Values={{'Off', 'On'}, [0 1]}
  Subsystem1 : Subsystem
  wires:
  Subsystem1/1(Out1) -> Data Store Write/1
  Mux/1 -> Subsystem1/1(In1)
  Constant/1 -> Mux/1
  Constant1/1 -> Mux/2
  Constant2/1 -> Mux/3

== system Autopilot_q_full_5may_new1/INITIALISE_PARAMS/If Action Subsystem/error_global ==
  ERROR_GLOBAL : DataStoreWrite  DataStoreName=error_global  DataStoreElements=error_global(1)#error_global(2)#error_global(3)#error_global(4)#error_global(5)#error_global(6)
  error_VX : Constant  Value=0
  error_VY : Constant  Value=0
  error_VZ : Constant  Value=0
  error_X : Constant  Value=0
  error_Y : Constant  Value=0
  error_Z : Constant  Value=0
  wires:
  error_Y/1 -> ERROR_GLOBAL/2
  error_VY/1 -> ERROR_GLOBAL/5
  error_X/1 -> ERROR_GLOBAL/1
  error_VZ/1 -> ERROR_GLOBAL/6
  error_Z/1 -> ERROR_GLOBAL/3
  error_VX/1 -> ERROR_GLOBAL/4

== system Autopilot_q_full_5may_new1/INITIALISE_PARAMS/If Action Subsystem/flags_global ==
  Fixed_wing_mode : Constant  Value=0
  Transition_mode : Constant  Value=0
  all_initial_check_ok : Constant
  brake_mode : Constant  Value=0
  default_mode : Constant
  fail_cruise_mode : Constant  Value=0
  fail_hover_mode : Constant  Value=0
  fail_safe_mode : Constant  Value=0
  fail_safe_mode_2 : Constant  Value=0
  fail_safe_mode_hover : Constant  Value=0
  fail_safe_mode_land : Constant  Value=0
  "flag store write " : DataStoreWrite  DataStoreName=flags_global  DataStoreElements=flags_global(1)#flags_global(2)#flags_global(3)#flags_global(4)#flags_global(5)#flags_global(6)#flags_global(7)#flags_global(8)#flags_global(9)#flags_global(10)#flags_global(11)#flags_global(12)#flags_global(13)#flags_global(14)#flags_global(15)#flags_global(16)#flags_global(17)#flags_global(18)#flags_global(19)#flags_global(20)#flags_global(21)#flags_global(22)#flags_global(23)#flags_global(24)#flags_global(25)#flags_global(26)
  flag_Forward_transition : Constant  Value=0
  flag_circle_mode : Constant  Value=0
  flag_initial_lift_off_hover : Constant
  flag_reverse_transition : Constant  Value=0
  flag_vertical_landing : Constant  Value=0
  flag_vertical_takeoff : Constant  Value=0
  one_time_initial_circle_mode : Constant
  one_time_initial_cruise_mode : Constant
  one_time_initial_forward_transition : Constant
  one_time_initial_hover_mode : Constant
  one_time_initial_lift_off_hover : Constant
  one_time_initial_reverse_transition : Constant
  one_time_initial_vertical_landing : Constant
  one_time_initial_vertical_takeoff : Constant
  quad_mode : Constant
  wires:
  one_time_initial_hover_mode/1 -> "flag store write "/18
  one_time_initial_vertical_landing/1 -> "flag store write "/21
  one_time_initial_reverse_transition/1 -> "flag store write "/26
  flag_reverse_transition/1 -> "flag store write "/24
  one_time_initial_forward_transition/1 -> "flag store write "/25
  one_time_initial_circle_mode/1 -> "flag store write "/20
  all_initial_check_ok/1 -> "flag store write "/1
  fail_hover_mode/1 -> "flag store write "/12
  Transition_mode/1 -> "flag store write "/4
  one_time_initial_lift_off_hover/1 -> "flag store write "/16
  fail_safe_mode_hover/1 -> "flag store write "/7
  brake_mode/1 -> "flag store write "/22
  one_time_initial_vertical_takeoff/1 -> "flag store write "/17
  flag_circle_mode/1 -> "flag store write "/13
  flag_initial_lift_off_hover/1 -> "flag store write "/10
  quad_mode/1 -> "flag store write "/3
  one_time_initial_cruise_mode/1 -> "flag store write "/19
  fail_safe_mode_2/1 -> "flag store write "/9
  flag_vertical_takeoff/1 -> "flag store write "/11
  fail_safe_mode/1 -> "flag store write "/6
  fail_cruise_mode/1 -> "flag store write "/14
  flag_Forward_transition/1 -> "flag store write "/23
  Fixed_wing_mode/1 -> "flag store write "/5
  default_mode/1 -> "flag store write "/2
  flag_vertical_landing/1 -> "flag store write "/15
  fail_safe_mode_land/1 -> "flag store write "/8

== system Autopilot_q_full_5may_new1/Wind_Model/System3/Subsystem1 ==
  i : Inport
  num : Inport  Port=2
  den : Inport  Port=3
  Derivative : Derivative
  Integrator : Integrator
  Integrator1 : Integrator
  MATLAB Function : MATLAB Function  TreatAsAtomicUnit=on
  Scope : Scope
  Scope1 : Scope
  Scope2 : Scope
  v_pert : Outport  VectorParamsAs1DForOutWhenUnconnected=off
  wires:
  Derivative/1 -> MATLAB Function/2(ii), Scope/1
  Integrator1/1 -> Scope2/1, v_pert/1, MATLAB Function/5(y)
  MATLAB Function/1(yyy) -> Integrator/1
  Integrator/1 -> Integrator1/1, MATLAB Function/6(yy)
  i/1 -> MATLAB Function/1(i), Derivative/1, Scope1/1
  num/1 -> MATLAB Function/3(num)
  den/1 -> MATLAB Function/4(den)

== system Autopilot_q_full_5may_new1/Wind_Model/System3/Subsystem4 ==
  i : Inport
  num : Inport  Port=2
  den : Inport  Port=3
  Integrator : Integrator
  MATLAB Function : MATLAB Function  TreatAsAtomicUnit=on
  Scope2 : Scope
  u_pert : Outport  VectorParamsAs1DForOutWhenUnconnected=off
  wires:
  den/1 -> MATLAB Function/3(den)
  num/1 -> MATLAB Function/2(num)
  i/1 -> MATLAB Function/1(i)
  Integrator/1 -> Scope2/1, u_pert/1, MATLAB Function/4(y)
  MATLAB Function/1(yy) -> Integrator/1

== system Autopilot_q_full_5may_new1/Wind_Model/System3/Subsystem5 ==
  i : Inport
  num : Inport  Port=2
  den : Inport  Port=3
  Band-Limited White Noise : simulink/Sources/Band-Limited White Noise  Cov=[0.001]  Ts=0.01  seed=[23341]
  Gain : Gain  Gain=0.01
  Integrator : Integrator
  Integrator1 : Integrator
  MATLAB Function : MATLAB Function  TreatAsAtomicUnit=on
  Scope2 : Scope
  Subtract : Sum  Inputs=+-
  w_pert : Outport  VectorParamsAs1DForOutWhenUnconnected=off
  wires:
  MATLAB Function/1(yyy) -> Integrator/1
  i/1 -> MATLAB Function/1(i), Subtract/1
  Integrator1/1 -> Scope2/1, w_pert/1, MATLAB Function/5(y)
  Integrator/1 -> Integrator1/1, MATLAB Function/6(yy)
  den/1 -> MATLAB Function/4(den)
  num/1 -> MATLAB Function/3(num)
  Subtract/1 -> Gain/1
  Gain/1 -> MATLAB Function/2(ii)
  Band-Limited White Noise/1 -> Subtract/2

== system Autopilot_q_full_5may_new1/AUTOPILOT /Autopilot Transition mode/Forward transition/Heading Controller ==
  "time " : Inport
  psi_d1 : Inport  Port=2
  Demux1 : Demux  Outputs=2
  Gain{,1..3} (4 alike) : Gain  Gain=57.3
  MATLAB Function : MATLAB Function  TreatAsAtomicUnit=on
  MATLAB Function5 : MATLAB Function  TreatAsAtomicUnit=on
  MATLAB Function6 : MATLAB Function  TreatAsAtomicUnit=on
  PID Controller : simulink/Continuous/PID Controller  Controller=PID  TimeDomain=Discrete-time  SampleTime=0.01  IntegratorMethod=Forward Euler  FilterMethod=Forward Euler  Form=Parallel  UseFilter=on  ControllerParametersSource=internal  P=0.33  I=0  D=0  N=100  InitialConditionSource=internal  InitialConditionForIntegrator=0  InitialConditionForFilter=0  ExternalReset=none  LimitOutput=off  UpperSaturationLimit=inf  LowerSaturationLimit=-inf  LinearizeAsGain=on  AntiWindupMode=none  Kb=1  TrackingMode=off  Kt=1  PParamMin=[]  PParamMax=[]  IParamMin=[]  IParamMax=[]  DParamMin=[]  DParamMax=[]  NParamMin=[]  NParamMax=[]  KbParamMin=[]  KbParamMax=[]  KtParamMin=[]  KtParamMax=[]  POutMin=[]  POutMax=[]  IOutMin=[]  IOutMax=[]  DOutMin=[]  DOutMax=[]  NOutMin=[]  NOutMax=[]  KbOutMin=[]  KbOutMax=[]  KtOutMin=[]  KtOutMax=[]  IntegratorOutMin=[]  IntegratorOutMax=[]  FilterOutMin=[]  FilterOutMax=[]  SumOutMin=[]  SumOutMax=[]  SumI1OutMin=[]  SumI1OutMax=[]  SumI2OutMin=[]  SumI2OutMax=[]  SumI3OutMin=[]  SumI3OutMax=[]  SumDOutMin=[]  SumDOutMax=[]  SaturationOutMin=[]  SaturationOutMax=[]  IntegratorContinuousStateAttributes=''  IntegratorStateMustResolveToSignalObject=off  IntegratorRTWStateStorageClass=Auto  FilterContinuousStateAttributes=''  FilterStateMustResolveToSignalObject=off  FilterRTWStateStorageClass=Auto  DifferentiatorICPrevScaledInput=0  DifferentiatorOutMin=[]  DifferentiatorOutMax=[]  FilterDiffOutCoefMin=[]  FilterDiffOutCoefMax=[]  SumDenOutMin=[]  SumDenOutMax=[]  SumNumOutMin=[]  SumNumOutMax=[]  ReciprocalOutMin=[]  ReciprocalOutMax=[]  DivideOutMin=[]  DivideOutMax=[]  TunerSelectOption=Transfer Function Based (PID Tuner App)
  PID Controller (2DOF)5 : simulink/Continuous/PID Controller (2DOF)  Controller=PID  TimeDomain=Discrete-time  SampleTime=0.01  IntegratorMethod=Forward Euler  FilterMethod=Forward Euler  Form=Parallel  UseFilter=on  ControllerParametersSource=internal  P=1.0  I=0.5  D=0  N=100  b=1  c=1  InitialConditionSource=internal  InitialConditionForIntegrator=0  InitialConditionForFilter=0  ExternalReset=none  LimitOutput=off  UpperSaturationLimit=inf  LowerSaturationLimit=-inf  LinearizeAsGain=on  AntiWindupMode=none  Kb=1  TrackingMode=off  Kt=1  PParamMin=[]  PParamMax=[]  IParamMin=[]  IParamMax=[]  DParamMin=[]  DParamMax=[]  NParamMin=[]  NParamMax=[]  bParamMin=[]  bParamMax=[]  cParamMin=[]  cParamMax=[]  KbParamMin=[]  KbParamMax=[]  KtParamMin=[]  KtParamMax=[]  POutMin=[]  POutMax=[]  IOutMin=[]  IOutMax=[]  DOutMin=[]  DOutMax=[]  NOutMin=[]  NOutMax=[]  bOutMin=[]  bOutMax=[]  cOutMin=[]  cOutMax=[]  KbOutMin=[]  KbOutMax=[]  KtOutMin=[]  KtOutMax=[]  IntegratorOutMin=[]  IntegratorOutMax=[]  FilterOutMin=[]  FilterOutMax=[]  SumOutMin=[]  SumOutMax=[]  Sum1OutMin=[]  Sum1OutMax=[]  Sum2OutMin=[]  Sum2OutMax=[]  Sum3OutMin=[]  Sum3OutMax=[]  SumI1OutMin=[]  SumI1OutMax=[]  SumI2OutMin=[]  SumI2OutMax=[]  SumI3OutMin=[]  SumI3OutMax=[]  SumDOutMin=[]  SumDOutMax=[]  SaturationOutMin=[]  SaturationOutMax=[]  IntegratorContinuousStateAttributes=''  IntegratorStateMustResolveToSignalObject=off  IntegratorRTWStateStorageClass=Auto  FilterContinuousStateAttributes=''  FilterStateMustResolveToSignalObject=off  FilterRTWStateStorageClass=Auto  DifferentiatorICPrevScaledInput=0  DifferentiatorOutMin=[]  DifferentiatorOutMax=[]  FilterDiffOutCoefMin=[]  FilterDiffOutCoefMax=[]  SumDenOutMin=[]  SumDenOutMax=[]  SumNumOutMin=[]  SumNumOutMax=[]  ReciprocalOutMin=[]  ReciprocalOutMax=[]  DivideOutMin=[]  DivideOutMax=[]  TunerSelectOption=Transfer Function Based (PID Tuner App)
  Scope : Scope  NumInputPorts=2
  Scope1 : Scope  NumInputPorts=2
  p,q,r,phi,theta,psi : DataStoreRead  DataStoreName=Plane_state_store  DataStoreElements=Plane_state_store(1,4:9)
  psi : DataStoreRead  DataStoreName=Plane_state_store  DataStoreElements=Plane_state_store(1,9)
  r : DataStoreRead  DataStoreName=Plane_state_store  DataStoreElements=Plane_state_store(1,6)
  u,v : DataStoreRead  DataStoreName=Plane_state_store  DataStoreElements=Plane_state_store(1,1:2)
  r_dot_d : Outport  VectorParamsAs1DForOutWhenUnconnected=off
  wires:
  u,v/1 -> Demux1/1
  MATLAB Function/1(psi_error) -> PID Controller/1
  Demux1/2 -> MATLAB Function5/3(v)
  r/1 -> Gain3/1, PID Controller (2DOF)5/2
  psi/1 -> MATLAB Function/2(psi), Gain1/1
  p,q,r,phi,theta,psi/1 -> MATLAB Function6/1(angular_state)
  MATLAB Function5/1(psi_d) -> Gain/1, MATLAB Function/1(psi_d)
  PID Controller/1 -> MATLAB Function6/2(psi_dot_d)
  MATLAB Function6/1(r_d) -> Gain2/1, PID Controller (2DOF)5/1
  Demux1/1 -> MATLAB Function5/2(u)
  PID Controller (2DOF)5/1 -> r_dot_d/1
  "time "/1 -> MATLAB Function5/1(t)
  psi_d1/1 -> MATLAB Function5/4("psi_d ")
  Gain/1 -> Scope/1
  Gain1/1 -> Scope/2
  Gain2/1 -> Scope1/1
  Gain3/1 -> Scope1/2

== system Autopilot_q_full_5may_new1/AUTOPILOT /Autopilot Transition mode/Forward transition/Pitch Controller ==
  a_x_d : Inport
  acc_d : Inport  Port=2
  Speed : Inport  Port=3
  stall speed : Inport  Port=4
  alpha_trim : Inport  Port=5
  Data Store Read1 : DataStoreRead  DataStoreName=Plane_state_store  DataStoreElements=Plane_state_store(:,:)
  Digital Clock : DigitalClock  SampleTime=0.01
  Gain7 : Gain  Gain=57.3
  Gain8 : Gain  Gain=57.3
  If : If  NumInputs=2  IfExpression=u1 > 5
  MATLAB Function3 : MATLAB Function  TreatAsAtomicUnit=on
  MATLAB Function4 : MATLAB Function  TreatAsAtomicUnit=on
  PID Controller (2DOF)3 : simulink/Continuous/PID Controller (2DOF)  Controller=PID  Form=Parallel  TimeDomain=Discrete-time  UseExternalTs=off  SampleTime=0.01  IntegratorMethod=Forward Euler  FilterMethod=Forward Euler  ControllerParametersSource=internal  P=12.0  I=6.0  D=0  UseFilter=on  N=100  b=1  c=1  TunerSelectOption=Transfer Function Based (PID Tuner App)  InitialConditionSource=internal  InitialConditionForIntegrator=0  InitialConditionForFilter=0  DifferentiatorICPrevScaledInput=0  ExternalReset=none  TrackingMode=off  Kt=1  LimitOutput=off  UpperSaturationLimit=inf  LowerSaturationLimit=-inf  LinearizeAsGain=on  AntiWindupMode=none  Kb=1  POutMin=[]  POutMax=[]  IOutMin=[]  IOutMax=[]  DOutMin=[]  DOutMax=[]  NOutMin=[]  NOutMax=[]  bOutMin=[]  bOutMax=[]  cOutMin=[]  cOutMax=[]  SumOutMin=[]  SumOutMax=[]  SaturationOutMin=[]  SaturationOutMax=[]  PParamMin=[]  PParamMax=[]  IParamMin=[]  IParamMax=[]  DParamMin=[]  DParamMax=[]  NParamMin=[]  NParamMax=[]  bParamMin=[]  bParamMax=[]  cParamMin=[]  cParamMax=[]  KbParamMin=[]  KbParamMax=[]  KtParamMin=[]  KtParamMax=[]  KbOutMin=[]  KbOutMax=[]  KtOutMin=[]  KtOutMax=[]  IntegratorOutMin=[]  IntegratorOutMax=[]  FilterOutMin=[]  FilterOutMax=[]  SumI1OutMin=[]  SumI1OutMax=[]  SumI2OutMin=[]  SumI2OutMax=[]  SumI3OutMin=[]  SumI3OutMax=[]  SumI4OutMin=[]  SumI4OutMax=[]  SumDOutMin=[]  SumDOutMax=[]  Sum1OutMin=[]  Sum1OutMax=[]  Sum2OutMin=[]  Sum2OutMax=[]  Sum3OutMin=[]  Sum3OutMax=[]  DifferentiatorOutMin=[]  DifferentiatorOutMax=[]  FilterDiffOutCoefMin=[]  FilterDiffOutCoefMax=[]  ReciprocalOutMin=[]  ReciprocalOutMax=[]  SumDenOutMin=[]  SumDenOutMax=[]  SumNumOutMin=[]  SumNumOutMax=[]  DivideOutMin=[]  DivideOutMax=[]  UdiffTsProdOutMin=[]  UdiffTsProdOutMax=[]  NTsProdOutMin=[]  NTsProdOutMax=[]  UintegralTsProdOutMin=[]  UintegralTsProdOutMax=[]  UngainTsProdOutMin=[]  UngainTsProdOutMax=[]  IntegratorContinuousStateAttributes=''  IntegratorStateMustResolveToSignalObject=off  IntegratorRTWStateStorageClass=Auto  FilterContinuousStateAttributes=''  FilterStateMustResolveToSignalObject=off  FilterRTWStateStorageClass=Auto  ParallelPVariant=InternalParameters  IdealPVariant=Disabled  IVariant=InternalParameters  DVariant=InternalParameters  bVariant=InternalParameters  cVariant=InternalParameters  IntegratorVariant=Discrete  SatVariant=Disabled  AWVariant=Passthrough  PCopyVariant=Disabled  TRVariant=Disabled  FdbkBlocksVariant=Forward  IdealPFdbkVariant=Disabled  SatFdbkVariant=Disabled  DerivativeFilterVariant=ForwardEulerFilter  NVariant=InternalParameters  NCopyVariant=Disabled  FilterICVariant=InternalICsFilter  IntegratorICVariant=InternalICs  ExternalResetVariant=Disabled  TRSumVariant=Passthrough  SumFdbkVariant=Disabled  SumVariant=Sum_PID  TsampFilterVariant=InternalTs  TsampNgainVariant=Passthrough  TsampIntegralVariant=Passthrough
  Scope7 : Scope  NumInputPorts=2
  Switch : Switch  Criteria=u2 > Threshold  Threshold=5.0
  alpha controller : Subsystem  TreatAsAtomicUnit=on
  ang_st1 : DataStoreRead  DataStoreName=Plane_state_store  DataStoreElements=Plane_state_store(1,4:9)
  "q " : DataStoreRead  DataStoreName=Plane_state_store  DataStoreElements=Plane_state_store(1,5)
  theta controller : Subsystem  TreatAsAtomicUnit=on
  Out1 : Outport  VectorParamsAs1DForOutWhenUnconnected=off
  wires:
  alpha controller/1(Output) -> MATLAB Function3/1(alpha_dot_d)
  PID Controller (2DOF)3/1 -> Out1/1
  Digital Clock/1 -> theta controller/1(time)
  MATLAB Function3/1(q_d) -> Switch/1
  ang_st1/1 -> MATLAB Function3/2(angular_state), MATLAB Function4/1(angular_state)
  Speed/1 -> If/1, Switch/2
  Gain8/1 -> Scope7/2
  MATLAB Function4/1(q_d) -> Switch/3
  theta controller/1(theta_dot) -> MATLAB Function4/2(theta_dot_d)
  Gain7/1 -> Scope7/1
  alpha_trim/1 -> theta controller/3(alpha_trim)
  a_x_d/1 -> theta controller/2(a_x_d)
  stall speed/1 -> If/2
  Data Store Read1/1 -> alpha controller/2(Plane_state)
  acc_d/1 -> alpha controller/1(acc_d)
  "q "/1 -> Gain8/1, PID Controller (2DOF)3/2
  Switch/1 -> Gain7/1, PID Controller (2DOF)3/1
  If/1 -> alpha controller/Action
  If/2 -> theta controller/Action
